simulink model "empc_motor_example"  (R2017a)
settings: Solver=ode45  StartTime=0.0  StopTime=20  RelTol=1e-3
values from neighbouring files (symbols this model uses):
  tau = tauam*pi*dshaft^3/16    (= 78.5398163397)    [motormodelexample.m]
libraries: mpclib x1, cstblocks x1
settings Model: ExtModeTrigMode=oneshot  ExtModeArmWhenConnect=off  Creator=The MathWorks, Inc.  LastModifiedBy=root
settings DataIOCC: SaveFormat=Array  SignalLoggingName=sigsOut
settings OptimizationCC: BooleanDataType=off  ExpressionDepthLimit=2147483647  InitFltsAndDblsToZero=on  LifeSpan=inf
settings DebuggingCC: SaveWithParameterizedLinksMsg=none  UnderspecifiedInitializationDetection=Classic  MergeDetectMultiDrivingBlocksExec=none  CheckExecutionContextPreStartOutputMsg=on  CheckExecutionContextRuntimeOutputMsg=on  SignalResolutionControl=TryResolveAllWithWarning  MultiTaskDSMMsg=warning  MultiTaskCondExecSysMsg=none  IntegerOverflowMsg=none  StateNameClashWarn=warning  SFUnexpectedBacktrackingDiag=warning  SFNoUnconditionalDefaultTransitionDiag=warning  SFExecutionAtInitializationDiag=none  IntegerSaturationMsg=none
settings HardwareCC: ProdBitPerPointer=32  ProdBitPerSizeT=32  ProdBitPerPtrDiffT=32  ProdLargestAtomicFloat=None  ProdIntDivRoundTo=Undefined  ProdEndianess=Unspecified  ProdWordSize=32  ProdHWDeviceType=32-bit Generic  TargetUnknown=on
settings ModelReferenceCC: PropagateSignalLabelsOutOfModel=off
settings GRTTargetCC: TargetFcnLib=ansi_tfl_tmw.mat  TargetLangStandard=C89/C90 (ANSI)  ModelReferenceCompliant=off  GeneratePreprocessorConditionals=Disable all  CombineOutputUpdateFcns=off  MatFileLogging=off  GRTInterface=on
settings ConfigComp: CovMetricSettings=dw  CovHtmlReporting=on  CovSaveCumulativeToWorkspaceVar=on  CovSaveSingleToWorkspaceVar=on  CovExternalEMLEnable=off  CovSFcnEnable=off

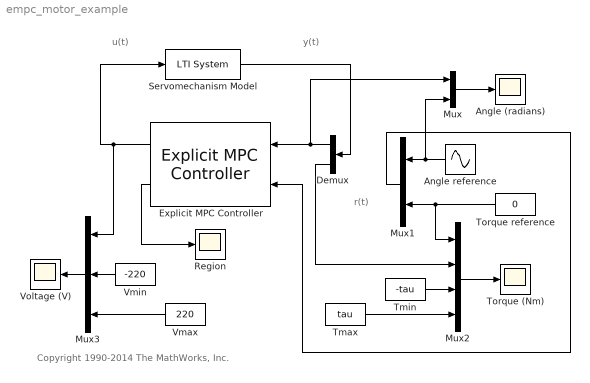
== system empc_motor_example ==
  note: u(t)
  note: y(t)
  note: r(t)
  note: Copyright 1990-2014 The MathWorks, Inc.
  Angle (radians) : Scope
  Angle reference : Sin  Amplitude=pi  Frequency=.4  SampleTime=0
  Demux : Demux  Outputs=2
  Explicit MPC Controller : mpclib/Explicit MPC Controller  SCDEnableBlockLinearizationSpecification=on  empcobj=mpcobjExplicit  is_multiple=0  enable_value=0  return_u0=off  md_inport=off  mv_inport=off  return_status=off  return_region=on  return_state=off  state_inport=off  BlockDataType=double  SampleTimeInherited=off  switch_inport=off
      settings: SourceProductName=Model Predictive Control Toolbox  SourceProductBaseCode=MP
  Mux : Mux  Inputs=2
  Mux1 : Mux  Inputs=2
  Mux2 : Mux
  Mux3 : Mux  Inputs=3
  Region : Scope
  Servomechanism Model : cstblocks/LTI System  sys=plant  IC=[]
  Tmax : Constant  Value=tau
  Tmin : Constant  Value=-tau
  Torque (Nm) : Scope
  Torque reference : Constant  Value=0
  Vmax : Constant  Value=220
  Vmin : Constant  Value=-220
  Voltage (V) : Scope
  wires:
  Servomechanism Model/1 -> Demux/1
  Mux/1 -> Angle (radians)/1
  Mux2/1 -> Torque (Nm)/1
  Demux/2 -> Mux2/2
  Mux1/1 -> Explicit MPC Controller/2
  Angle reference/1 -> Mux1/1, Mux/2
  Demux/1 -> Mux/1, Explicit MPC Controller/1
  Mux3/1 -> Voltage (V)/1
  Vmin/1 -> Mux3/2
  Vmax/1 -> Mux3/3
  Tmin/1 -> Mux2/3
  Tmax/1 -> Mux2/4
  Torque reference/1 -> Mux1/2, Mux2/1
  Explicit MPC Controller/1 -> Mux3/1, Servomechanism Model/1
  Explicit MPC Controller/2 -> Region/1
